simulink model "stateSpace0"  (R2020a)
settings: Solver=VariableStepAuto  StartTime=0.0  StopTime=10  RelTol=1e-3  EnableMultiTasking=on
settings Model: Creator=bkhusain  LastModifiedBy=mmarathe
settings DataIOCC: LimitDataPoints=on  MaxDataPoints=10000
settings OptimizationCC: LifeSpan=inf
settings DebuggingCC: AllowSymbolicDim=off  SFUnexpectedBacktrackingDiag=warning  SFNoUnconditionalDefaultTransitionDiag=warning  SFExecutionAtInitializationDiag=none  ArithmeticOperatorsInVariantConditions=warning
settings SFSimCC: SimUseLocalCustomCode=off  CustomCodeUndefinedFunction=UseInterfaceOnly
settings RTWCC: RTWUseLocalCustomCode=off
settings CodeAppCC: StateflowObjectComments=on
settings GRTTargetCC: TargetLangStandard=C89/C90 (ANSI)
settings ConfigComp: CovMetricSettings=dw  CovHtmlReporting=on  CovSaveCumulativeToWorkspaceVar=on  CovSaveSingleToWorkspaceVar=on  CovExternalEMLEnable=off  CovSFcnEnable=off
settings SimscapeCC: SimscapeLogType=all  SimscapeLogSimulationStatistics=on  SimscapeLogDataHistory=10000

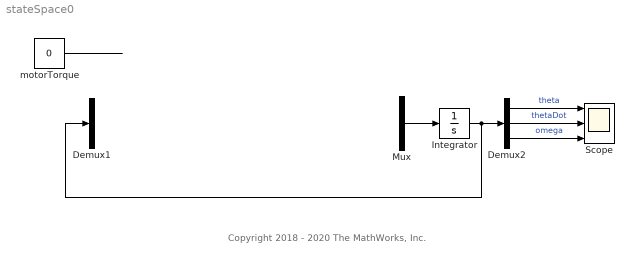
== system stateSpace0 ==
  note: Copyright 2018 - 2020 The MathWorks, Inc.
  Demux1 : Demux  Outputs=3
  Demux2 : Demux  Outputs=3
  Integrator : Integrator
  Mux : Mux  Inputs=3
  Scope : Scope  NumInputPorts=3
  motorTorque : Constant  Value=0
  wires:
  Demux2/1 -> Scope/1  "theta"
  Demux2/3 -> Scope/3  "omega"
  Integrator/1 -> Demux2/1, Demux1/1
  Demux2/2 -> Scope/2  "thetaDot"
  motorTorque/1 -> ?
  ? -> Mux/2  "thetaDot"
  Mux/1 -> Integrator/1
  ? -> Mux/1  "thetaDdot"
  ? -> Mux/3  "omegaDot"
